simulink model "DecisionLogic"  (R2024b)
settings: Solver=VariableStepAuto  StartTime=0.0  StopTime=scenario.StopTime  FixedStep=0.001  RelTol=1e-8  EnableMultiTasking=on
undefined symbols (not defined in the file or in its folder): maxMIOLeadDistance, posSelector, Ts, velSelector
settings Model: Creator=The MathWorks, Inc.  LastModifiedBy=Pranith
settings SolverCC: ZeroCrossAlgorithm=Adaptive  AlgebraicLoopSolver=TrustRegion  PositivePriorityOrder=on  AutoInsertRateTranBlk=on  InsertRTBMode=Always  DecoupledContinuousIntegration=on  MinimalZcImpactIntegration=on  MaxZcPerStep=1
settings DataIOCC: SaveOutput=off  SaveTime=off  ReturnWorkspaceOutputs=off
settings DebuggingCC: IntegerOverflowMsg=none  ParameterPrecisionLossMsg=none  UnconnectedInputMsg=warning  UnconnectedOutputMsg=warning  UnconnectedLineMsg=warning  PregeneratedLibrarySubsystemCodeDiagnostic=none  SubsystemReferenceDiagnosticForUnitTest=warning  IntegerSaturationMsg=none  ArithmeticOperatorsInVariantConditions=warning
settings HardwareCC: ProdLongLongMode=on
settings ModelReferenceCC: EnableRefExpFcnMdlSchedulingChecks=on
settings SFSimCC: SimUseLocalCustomCode=off
settings RTWCC: GenerateReport=on  RTWUseLocalCustomCode=off  LaunchReport=on  GPUComputeCapability=3.5  DLArmComputeVersion=19.05
settings ConfigComp: CovScope=ReferencedModels  CovIncludeTopModel=off

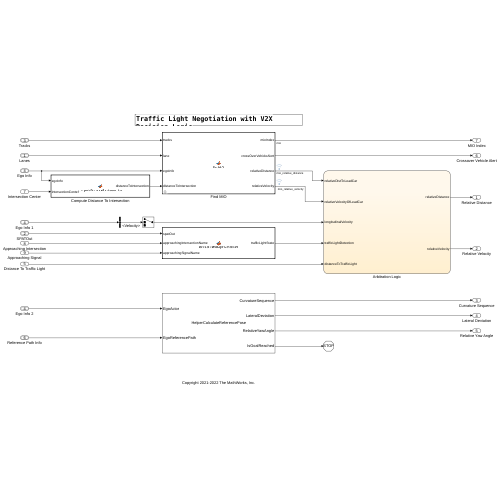
[thumbnail: Simulink's stored preview of the top-level diagram]
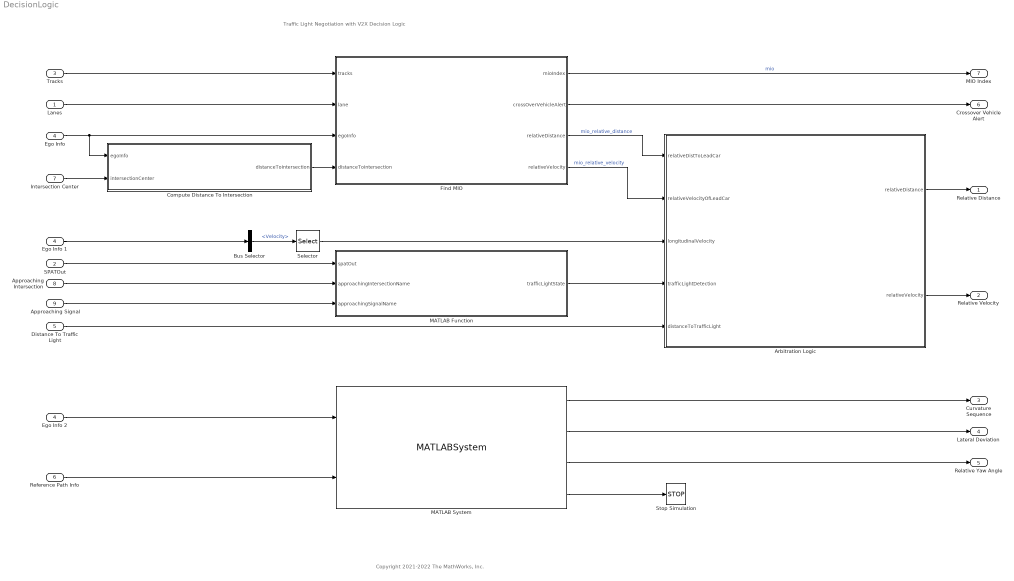
== system DecisionLogic ==
  note: Traffic Light Negotiation with V2X Decision Logic
  note: Copyright 2021-2022 The MathWorks, Inc.
  Lanes : Inport  OutDataTypeStr=Bus: LaneSensor
  SPATOut : Inport  Port=2  OutDataTypeStr=Bus: BusSPAT  BusOutputAsStruct=on
  Tracks : Inport  Port=3  OutDataTypeStr=Bus: BusMultiObjectTracker  BusOutputAsStruct=on
  "Ego Info " : Inport  Port=4  OutDataTypeStr=Bus: BusVehiclePose  SampleTime=[0.10000000000000001,0]
  Distance To Traffic Light : Inport  Port=5  OutDataTypeStr=double  PortDimensions=1  SampleTime=[0.10000000000000001,0]
  "Reference Path Info " : Inport  Port=6  OutDataTypeStr=Bus: ReferencePathInfo  PortDimensions=1  SampleTime=[0.10000000000000001,0]  BusOutputAsStruct=on
  Intersection Center : Inport  Port=7  OutDataTypeStr=double  PortDimensions=3  SampleTime=[0.10000000000000001,0]
  Approaching Intersection : Inport  Port=8  OutDataTypeStr=string
  Approaching Signal : Inport  Port=9  OutDataTypeStr=string
  Arbitration Logic : Stateflow chart  TreatAsAtomicUnit=on  SystemSampleTime=Ts
  Bus Selector : BusSelector  OutputSignals=Velocity
  Compute Distance To Intersection : MATLAB Function  TreatAsAtomicUnit=on
  Ego Info 1 : InportShadow  Port=4  OutDataTypeStr=Bus: BusVehiclePose  SampleTime=[0.10000000000000001,0]
  Ego Info 2 : InportShadow  Port=4  OutDataTypeStr=Bus: BusVehiclePose  SampleTime=[0.10000000000000001,0]
  Find MIO : MATLAB Function  TreatAsAtomicUnit=on  SystemSampleTime=Ts  mask{maxDistance=maxMIOLeadDistance, posSelector=posSelector, velSelector=velSelector}
      mask prompts: maxDistance "Maximum lead distance"; posSelector "Track Position Selector"; velSelector "Track Velocity Selector"
  MATLAB Function : MATLAB Function  TreatAsAtomicUnit=on
  MATLAB System : MATLABSystem  System=HelperCalculateReferencePose  PredictionHorizon=PredictionHorizon  DistanceFromCGToRear=lr  SampleTime=0.1  SimulateUsing=Code generation
      mask Type: HelperCalculateReferencePose
      mask Display:
      | disp('HelperCalculateReferencePose');
      | port_label('input',1,'EgoActor');
      | port_label('input',2,'EgoReferencePath');
      | port_label('output',1,'CurvatureSequence');
      | port_label('output',2,'LateralDeviation');
      | port_label('output',3,'RelativeYawAngle');
      | port_label('output',4,'IsGoalReached');
  Selector : Selector  InputPortWidth=3  IndexOptions=Index vector (dialog)  Indices=[1]  OutputSizes=1
  Stop Simulation : Stop
  Relative Distance : Outport  OutDataTypeStr=double  PortDimensions=1  SampleTime=[0.10000000000000001,0]  VectorParamsAs1DForOutWhenUnconnected=off
  Relative Velocity : Outport  Port=2  OutDataTypeStr=double  PortDimensions=1  SampleTime=[0.10000000000000001,0]  VectorParamsAs1DForOutWhenUnconnected=off
  Curvature Sequence : Outport  Port=3
  Lateral Deviation : Outport  Port=4
  Relative Yaw Angle : Outport  Port=5
  Crossover Vehicle Alert : Outport  Port=6
  MIO Index : Outport  Port=7
  wires:
  Lanes/1 -> Find MIO/2(lane)
  Arbitration Logic/1(relativeDistance) -> Relative Distance/1
  Arbitration Logic/2(relativeVelocity) -> Relative Velocity/1
  SPATOut/1 -> MATLAB Function/1(spatOut)
  Distance To Traffic Light/1 -> Arbitration Logic/5(distanceToTrafficLight)
  Find MIO/3(relativeDistance) -> Arbitration Logic/1(relativeDistToLeadCar)  "mio_relative_distance"
  Find MIO/4(relativeVelocity) -> Arbitration Logic/2(relativeVelocityOfLeadCar)  "mio_relative_velocity"
  Find MIO/1(mioIndex) -> MIO Index/1  "mio"
  Tracks/1 -> Find MIO/1(tracks)
  MATLAB Function/1(trafficLightState) -> Arbitration Logic/4(trafficLightDetection)
  Find MIO/2(crossOverVehicleAlert) -> Crossover Vehicle Alert/1
  Bus Selector/1 -> Selector/1  "<Velocity>"
  Selector/1 -> Arbitration Logic/3(longitudinalVelocity)
  Approaching Intersection/1 -> MATLAB Function/2(approachingIntersectionName)
  Approaching Signal/1 -> MATLAB Function/3(approachingSignalName)
  Compute Distance To Intersection/1(distanceToIntersection) -> Find MIO/4(distanceToIntersection)
  Intersection Center/1 -> Compute Distance To Intersection/2(intersectionCenter)
  "Ego Info "/1 -> Find MIO/3(egoInfo), Compute Distance To Intersection/1(egoInfo)
  Ego Info 1/1 -> Bus Selector/1
  "Reference Path Info "/1 -> MATLAB System/2
  Ego Info 2/1 -> MATLAB System/1
  MATLAB System/1 -> Curvature Sequence/1
  MATLAB System/2 -> Lateral Deviation/1
  MATLAB System/3 -> Relative Yaw Angle/1
  MATLAB System/4 -> Stop Simulation/1

== matlab function DecisionLogic/Compute Distance To Intersection ==
  data: egoInfo input; intersectionCenter input; distanceToIntersection output
function distanceToIntersection = computeDistanceToIntersection(egoInfo,intersectionCenter)

currentEgoPose = [0 0 0];
currentEgoPose = egoInfo.Position;
distanceToIntersection = double(sqrt((intersectionCenter(1)- ...
    currentEgoPose(1))^2 + (intersectionCenter(2)- currentEgoPose(2))^2));

end

== matlab function DecisionLogic/MATLAB Function ==
  data: spatOut input; trafficLightState output; approachingIntersectionName input; approachingSignalName input
function trafficLightState = extractTrafficLightDetection(spatOut,approachingIntersectionName,approachingSignalName)
    % approachingIntersectionName = "TrafficLightGroup_1";
    % approachingSignalName = "TrafficLight_1";
    trafficLightState = -1;
    coder.extrinsic("helperGetTrafficLightDetection")
    trafficLightState = helperGetTrafficLightDetection(spatOut,approachingIntersectionName,approachingSignalName);
end

== stateflow chart DecisionLogic/Arbitration Logic ==
  state OnEntry
    entry:
    relativeDistance = relativeDistToLeadCar;
    relativeVelocity = relativeVelocityOfLeadCar;
  state OnRedAndYellowLightDetection
    entry:
    relativeDistance = min(relativeDistToLeadCar,distanceToTrafficLight);
    relativeVelocity = min(relativeVelocityOfLeadCar,longitudinalVelocity);
  (default) -> OnEntry
  OnEntry -> OnEntry [order 2] : [hasChanged(relativeDistToLeadCar)]
  OnRedAndYellowLightDetection -> OnEntry [order 1] : [trafficLightDetection==Green || trafficLightDetection == NoDetections  ]
  OnEntry -> OnRedAndYellowLightDetection [order 1] : [(trafficLightDetection==Red || trafficLightDetection==Yellow) && distanceToTrafficLight ~= inf]
  OnRedAndYellowLightDetection -> OnRedAndYellowLightDetection [order 2] : [hasChanged(relativeDistToLeadCar)]
  OnRedAndYellowLightDetection -> OnRedAndYellowLightDetection [order 3] : [hasChanged(distanceToTrafficLight)]
  data: relativeDistance output; relativeDistToLeadCar input; relativeVelocityOfLeadCar input; longitudinalVelocity input; trafficLightDetection input; distanceToTrafficLight input; relativeVelocity output; Green local =2; Red local =0; Yellow local =1; NoDetections local =-1

== matlab function DecisionLogic/Find MIO ==
  data: mioIndex output; crossOverVehicleAlert output; tracks input; relativeDistance output size=[1 1] [-inf..inf]; relativeVelocity output size=[1 1] [-inf..inf]; lane input; egoInfo input; maxDistance parameter; distanceToIntersection input; posSelector parameter; velSelector parameter
function [mioIndex,crossOverVehicleAlert,relativeDistance,relativeVelocity] = findMIO(tracks, lane, egoInfo, maxDistance,distanceToIntersection,posSelector, velSelector)
% This function finds the MIO: Which satisfies all the criteria below:
% * Within the ego car's lane.
% * In front of the ego car.
% * Approaching the ego from the left or right at intersection

% Copyright 2021 The MathWorks, Inc.
[relativeDistance,relativeVelocity,mioIndex,crossOverVehicleAlert] = helperFindMIO(tracks, lane, egoInfo,maxDistance,distanceToIntersection,posSelector,velSelector);
